simulink model "gm_UZ_EnDat"  (R2023b)
settings: Solver=FixedStepDiscrete  StartTime=0  StopTime=0.002  RelTol=1e-3
model workspace (MAT data in the model file):
  Select = 0
libraries: hdlsllib x314, hdlmdlgenlib x10, simulink x7, simulink_extras x3
(part 2 of 7)

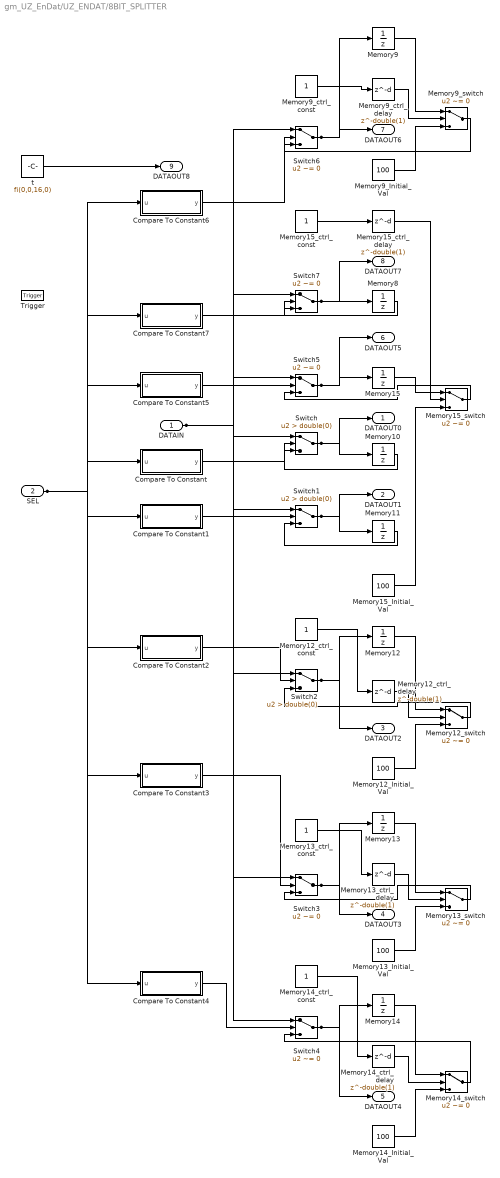
== system gm_UZ_EnDat/UZ_ENDAT/8BIT_SPLITTER ==
  DATAIN : Inport  OutDataTypeStr=uint16  PortDimensions=1
  SEL : Inport  Port=2  OutDataTypeStr=fixdt(0, 4, 0)  PortDimensions=1
  Trigger : TriggerPort  TriggerType=falling  VariantControl=(inherit)  OutputDataType=int8  InitialTriggerSignalState=positive  PortDimensions=1  OutDataTypeStr=boolean
  Compare To Constant : Subsystem  mask(Compare To Constant){relop===, const=double(0), OutDataTypeStr=boolean, ZeroCross=on}
      mask prompts: relop "Simulink:masks:Operator_MP"; const "Simulink:masks:ConstantValue_MP"; OutDataTypeStr "Simulink:masks:OutputDataType_MP"; ZeroCross "Simulink:masks:EnableZerocrossingDetection_MP"
      mask help: Simulink:masks:CompareToConstant_MD
      mask TypeOptions relop: == | ~= | < | <= | >= | >
      mask TypeOptions OutDataTypeStr: Simulink:masks:uint8 | Simulink:masks:boolean
      mask Callback ZeroCross: sl('zeroCrossEnable', gcbh);
      mask Display: disp(str)
  Compare To Constant1 : Subsystem  mask(Compare To Constant){relop===, const=double(1), OutDataTypeStr=boolean, ZeroCross=on}
      mask prompts: relop "Simulink:masks:Operator_MP"; const "Simulink:masks:ConstantValue_MP"; OutDataTypeStr "Simulink:masks:OutputDataType_MP"; ZeroCross "Simulink:masks:EnableZerocrossingDetection_MP"
      mask help: Simulink:masks:CompareToConstant_MD
      mask init:
      | OutDataTypeStr = 'boolean';
      | ZeroCross = 'on';
      | blkName = 'UZ_EnDat/UZ_ENDAT/8BIT_SPLITTER/Compare\nTo Constant1';
      | const = double(1);
      | const_str = '1';
      | const_val = double(1);
      | relop = '==';
      | setValue = 'boolean';
      | str = '== 1';
      mask TypeOptions relop: == | ~= | < | <= | >= | >
      mask TypeOptions OutDataTypeStr: Simulink:masks:uint8 | Simulink:masks:boolean
      mask Callback ZeroCross: sl('zeroCrossEnable', gcbh);
      mask Display: disp(str)
  Compare To Constant2 : Subsystem  mask(Compare To Constant){relop===, const=double(2), OutDataTypeStr=boolean, ZeroCross=on}
      mask prompts: relop "Simulink:masks:Operator_MP"; const "Simulink:masks:ConstantValue_MP"; OutDataTypeStr "Simulink:masks:OutputDataType_MP"; ZeroCross "Simulink:masks:EnableZerocrossingDetection_MP"
      mask help: Simulink:masks:CompareToConstant_MD
      mask init:
      | OutDataTypeStr = 'boolean';
      | ZeroCross = 'on';
      | blkName = 'UZ_EnDat/UZ_ENDAT/8BIT_SPLITTER/Compare\nTo Constant2';
      | const = double(2);
      | const_str = '2';
      | const_val = double(2);
      | relop = '==';
      | setValue = 'boolean';
      | str = '== 2';
      mask TypeOptions relop: == | ~= | < | <= | >= | >
      mask TypeOptions OutDataTypeStr: Simulink:masks:uint8 | Simulink:masks:boolean
      mask Callback ZeroCross: sl('zeroCrossEnable', gcbh);
      mask Display: disp(str)
  Compare To Constant3 : Subsystem  mask(Compare To Constant){relop===, const=double(3), OutDataTypeStr=boolean, ZeroCross=on}
      mask prompts: relop "Simulink:masks:Operator_MP"; const "Simulink:masks:ConstantValue_MP"; OutDataTypeStr "Simulink:masks:OutputDataType_MP"; ZeroCross "Simulink:masks:EnableZerocrossingDetection_MP"
      mask help: Simulink:masks:CompareToConstant_MD
      mask init:
      | OutDataTypeStr = 'boolean';
      | ZeroCross = 'on';
      | blkName = 'UZ_EnDat/UZ_ENDAT/8BIT_SPLITTER/Compare\nTo Constant3';
      | const = double(3);
      | const_str = '3';
      | const_val = double(3);
      | relop = '==';
      | setValue = 'boolean';
      | str = '== 3';
      mask TypeOptions relop: == | ~= | < | <= | >= | >
      mask TypeOptions OutDataTypeStr: Simulink:masks:uint8 | Simulink:masks:boolean
      mask Callback ZeroCross: sl('zeroCrossEnable', gcbh);
      mask Display: disp(str)
  Compare To Constant4 : Subsystem  mask(Compare To Constant){relop===, const=double(4), OutDataTypeStr=boolean, ZeroCross=on}
      mask prompts: relop "Simulink:masks:Operator_MP"; const "Simulink:masks:ConstantValue_MP"; OutDataTypeStr "Simulink:masks:OutputDataType_MP"; ZeroCross "Simulink:masks:EnableZerocrossingDetection_MP"
      mask help: Simulink:masks:CompareToConstant_MD
      mask init:
      | OutDataTypeStr = 'boolean';
      | ZeroCross = 'on';
      | blkName = 'UZ_EnDat/UZ_ENDAT/8BIT_SPLITTER/Compare\nTo Constant4';
      | const = double(4);
      | const_str = '4';
      | const_val = double(4);
      | relop = '==';
      | setValue = 'boolean';
      | str = '== 4';
      mask TypeOptions relop: == | ~= | < | <= | >= | >
      mask TypeOptions OutDataTypeStr: Simulink:masks:uint8 | Simulink:masks:boolean
      mask Callback ZeroCross: sl('zeroCrossEnable', gcbh);
      mask Display: disp(str)
  Compare To Constant5 : Subsystem  mask(Compare To Constant){relop===, const=double(5), OutDataTypeStr=boolean, ZeroCross=on}
      mask prompts: relop "Simulink:masks:Operator_MP"; const "Simulink:masks:ConstantValue_MP"; OutDataTypeStr "Simulink:masks:OutputDataType_MP"; ZeroCross "Simulink:masks:EnableZerocrossingDetection_MP"
      mask help: Simulink:masks:CompareToConstant_MD
      mask init:
      | OutDataTypeStr = 'boolean';
      | ZeroCross = 'on';
      | blkName = 'UZ_EnDat/UZ_ENDAT/8BIT_SPLITTER/Compare\nTo Constant5';
      | const = double(5);
      | const_str = '5';
      | const_val = double(5);
      | relop = '==';
      | setValue = 'boolean';
      | str = '== 5';
      mask TypeOptions relop: == | ~= | < | <= | >= | >
      mask TypeOptions OutDataTypeStr: Simulink:masks:uint8 | Simulink:masks:boolean
      mask Callback ZeroCross: sl('zeroCrossEnable', gcbh);
      mask Display: disp(str)
  Compare To Constant6 : Subsystem  mask(Compare To Constant){relop===, const=double(6), OutDataTypeStr=boolean, ZeroCross=on}
      mask prompts: relop "Simulink:masks:Operator_MP"; const "Simulink:masks:ConstantValue_MP"; OutDataTypeStr "Simulink:masks:OutputDataType_MP"; ZeroCross "Simulink:masks:EnableZerocrossingDetection_MP"
      mask help: Simulink:masks:CompareToConstant_MD
      mask init:
      | OutDataTypeStr = 'boolean';
      | ZeroCross = 'on';
      | blkName = 'UZ_EnDat/UZ_ENDAT/8BIT_SPLITTER/Compare\nTo Constant6';
      | const = double(6);
      | const_str = '6';
      | const_val = double(6);
      | relop = '==';
      | setValue = 'boolean';
      | str = '== 6';
      mask TypeOptions relop: == | ~= | < | <= | >= | >
      mask TypeOptions OutDataTypeStr: Simulink:masks:uint8 | Simulink:masks:boolean
      mask Callback ZeroCross: sl('zeroCrossEnable', gcbh);
      mask Display: disp(str)
  Compare To Constant7 : Subsystem  mask(Compare To Constant){relop===, const=double(7), OutDataTypeStr=boolean, ZeroCross=on}
      mask prompts: relop "Simulink:masks:Operator_MP"; const "Simulink:masks:ConstantValue_MP"; OutDataTypeStr "Simulink:masks:OutputDataType_MP"; ZeroCross "Simulink:masks:EnableZerocrossingDetection_MP"
      mask help: Simulink:masks:CompareToConstant_MD
      mask init:
      | OutDataTypeStr = 'boolean';
      | ZeroCross = 'on';
      | blkName = 'UZ_EnDat/UZ_ENDAT/8BIT_SPLITTER/Compare\nTo Constant7';
      | const = double(7);
      | const_str = '7';
      | const_val = double(7);
      | relop = '==';
      | setValue = 'boolean';
      | str = '== 7';
      mask TypeOptions relop: == | ~= | < | <= | >= | >
      mask TypeOptions OutDataTypeStr: Simulink:masks:uint8 | Simulink:masks:boolean
      mask Callback ZeroCross: sl('zeroCrossEnable', gcbh);
      mask Display: disp(str)
  Memory10 : UnitDelay  SampleTime=-1
  Memory11 : UnitDelay  SampleTime=-1
  Memory{9,12..15} (5 alike) : UnitDelay  InitialCondition=double(0)  SampleTime=-1
  Memory12_Initial_Val : Constant  Value=100  OutDataTypeStr=uint16  SampleTime=-1
  Memory12_ctrl_const : Constant  OutDataTypeStr=boolean  SampleTime=-1
  Memory12_ctrl_delay : Delay  DelayLength=double(1)  InitialCondition=0
  Memory12_switch : Switch  Criteria=u2 ~= 0  Threshold=double(0)  OutDataTypeStr=uint16  SaturateOnIntegerOverflow=off  InputSameDT=off
  Memory13_Initial_Val : Constant  Value=100  OutDataTypeStr=uint16  SampleTime=-1
  Memory13_ctrl_const : Constant  OutDataTypeStr=boolean  SampleTime=-1
  Memory13_ctrl_delay : Delay  DelayLength=double(1)  InitialCondition=0
  Memory13_switch : Switch  Criteria=u2 ~= 0  Threshold=double(0)  OutDataTypeStr=uint16  SaturateOnIntegerOverflow=off  InputSameDT=off
  Memory14_Initial_Val : Constant  Value=100  OutDataTypeStr=uint16  SampleTime=-1
  Memory14_ctrl_const : Constant  OutDataTypeStr=boolean  SampleTime=-1
  Memory14_ctrl_delay : Delay  DelayLength=double(1)  InitialCondition=0
  Memory14_switch : Switch  Criteria=u2 ~= 0  Threshold=double(0)  OutDataTypeStr=uint16  SaturateOnIntegerOverflow=off  InputSameDT=off
  Memory15_Initial_Val : Constant  Value=100  OutDataTypeStr=uint16  SampleTime=-1
  Memory15_ctrl_const : Constant  OutDataTypeStr=boolean  SampleTime=-1
  Memory15_ctrl_delay : Delay  DelayLength=double(1)  InitialCondition=0
  Memory15_switch : Switch  Criteria=u2 ~= 0  Threshold=double(0)  OutDataTypeStr=uint16  SaturateOnIntegerOverflow=off  InputSameDT=off
  Memory8 : UnitDelay  SampleTime=-1
  Memory9_Initial_Val : Constant  Value=100  OutDataTypeStr=uint16  SampleTime=-1
  Memory9_ctrl_const : Constant  OutDataTypeStr=boolean  SampleTime=-1
  Memory9_ctrl_delay : Delay  DelayLength=double(1)  InitialCondition=0
  Memory9_switch : Switch  Criteria=u2 ~= 0  Threshold=double(0)  OutDataTypeStr=uint16  SaturateOnIntegerOverflow=off  InputSameDT=off
  Switch : Switch  Criteria=u2 > Threshold  Threshold=double(0)  OutDataTypeStr=uint16  SaturateOnIntegerOverflow=off  InputSameDT=off
  Switch1 : Switch  Criteria=u2 > Threshold  Threshold=double(0)  OutDataTypeStr=uint16  SaturateOnIntegerOverflow=off  InputSameDT=off
  Switch2 : Switch  Criteria=u2 > Threshold  Threshold=double(0)  OutDataTypeStr=uint16  SaturateOnIntegerOverflow=off  InputSameDT=off
  Switch{3..6} (4 alike) : Switch  Criteria=u2 ~= 0  Threshold=double(0)  OutDataTypeStr=uint16  SaturateOnIntegerOverflow=off  InputSameDT=off
  Switch7 : Switch  Criteria=u2 ~= 0  Threshold=double(0)  OutDataTypeStr=int8  SaturateOnIntegerOverflow=off  InputSameDT=off
  t : Constant  Value=fi(0,0,16,0)  OutDataTypeStr=uint16  SampleTime=-1
  DATAOUT0 : Outport  InitialOutput=0
  DATAOUT1 : Outport  Port=2  InitialOutput=0
  DATAOUT2 : Outport  Port=3  InitialOutput=0
  DATAOUT3 : Outport  Port=4  InitialOutput=0
  DATAOUT4 : Outport  Port=5  InitialOutput=0
  DATAOUT5 : Outport  Port=6  InitialOutput=0
  DATAOUT6 : Outport  Port=7  InitialOutput=0
  DATAOUT7 : Outport  Port=8  InitialOutput=0
  DATAOUT8 : Outport  Port=9  InitialOutput=0
  wires:
  DATAIN/1 -> Switch/1, Switch1/1, Switch2/1, Switch3/1, Switch4/1, Switch5/1, Switch6/1, Switch7/1
  SEL/1 -> Compare To Constant6/1(u), Compare To Constant7/1(u), Compare To Constant5/1(u), Compare To Constant4/1(u), Compare To Constant2/1(u), Compare To Constant1/1(u), Compare To Constant/1(u), Compare To Constant3/1(u)
  Switch/1 -> DATAOUT0/1, Memory10/1
  Switch1/1 -> DATAOUT1/1, Memory11/1
  Switch2/1 -> DATAOUT2/1, Memory12/1
  Switch3/1 -> DATAOUT3/1, Memory13/1
  Switch4/1 -> DATAOUT4/1, Memory14/1
  Switch5/1 -> DATAOUT5/1, Memory15/1
  Switch6/1 -> DATAOUT6/1, Memory9/1
  Switch7/1 -> DATAOUT7/1, Memory8/1
  t/1 -> DATAOUT8/1
  Compare To Constant7/1(y) -> Switch7/2
  Memory8/1 -> Switch7/3
  Compare To Constant/1(y) -> Switch/2
  Memory10/1 -> Switch/3
  Compare To Constant1/1(y) -> Switch1/2
  Memory11/1 -> Switch1/3
  Memory12/1 -> Memory12_switch/1
  Memory12_ctrl_delay/1 -> Memory12_switch/2
  Memory12_Initial_Val/1 -> Memory12_switch/3
  Compare To Constant2/1(y) -> Switch2/2
  Memory12_switch/1 -> Switch2/3
  Memory13/1 -> Memory13_switch/1
  Memory13_ctrl_delay/1 -> Memory13_switch/2
  Memory13_Initial_Val/1 -> Memory13_switch/3
  Compare To Constant3/1(y) -> Switch3/2
  Memory13_switch/1 -> Switch3/3
  Memory14/1 -> Memory14_switch/1
  Memory14_ctrl_delay/1 -> Memory14_switch/2
  Memory14_Initial_Val/1 -> Memory14_switch/3
  Compare To Constant4/1(y) -> Switch4/2
  Memory14_switch/1 -> Switch4/3
  Memory15/1 -> Memory15_switch/1
  Memory15_ctrl_delay/1 -> Memory15_switch/2
  Memory15_Initial_Val/1 -> Memory15_switch/3
  Compare To Constant5/1(y) -> Switch5/2
  Memory15_switch/1 -> Switch5/3
  Memory9/1 -> Memory9_switch/1
  Memory9_ctrl_delay/1 -> Memory9_switch/2
  Memory9_Initial_Val/1 -> Memory9_switch/3
  Compare To Constant6/1(y) -> Switch6/2
  Memory9_switch/1 -> Switch6/3
  Memory12_ctrl_const/1 -> Memory12_ctrl_delay/1
  Memory13_ctrl_const/1 -> Memory13_ctrl_delay/1
  Memory14_ctrl_const/1 -> Memory14_ctrl_delay/1
  Memory15_ctrl_const/1 -> Memory15_ctrl_delay/1
  Memory9_ctrl_const/1 -> Memory9_ctrl_delay/1

== system gm_UZ_EnDat/UZ_ENDAT/CLKCNTER_ACT ==
  CLK : Inport  OutDataTypeStr=boolean  PortDimensions=1  SampleTime=1e-08
  CLK2CNT : Inport  Port=2  OutDataTypeStr=boolean  PortDimensions=1  SampleTime=1e-08
  ResetCNT : Inport  Port=3  OutDataTypeStr=boolean  PortDimensions=1  SampleTime=1e-08
  Delay1 : Delay  DelayLength=double(1)  InitialCondition=0  SampleTime=1e-08
  Positional_Counter : Subsystem
  SetZero32modified : Subsystem
  CNT : Outport  SampleTime=1e-08
  wires:
  Positional_Counter/1(divider) -> SetZero32modified/1(valin)
  CLK/1 -> SetZero32modified/Trigger
  ResetCNT/1 -> SetZero32modified/2(setzero)
  CLK2CNT/1 -> Positional_Counter/Trigger
  SetZero32modified/1(valueout) -> Delay1/1
  Delay1/1 -> Positional_Counter/1(valueout), CNT/1

== system gm_UZ_EnDat/UZ_ENDAT/CLKCNTER_NOSTOP ==
  CLK : Inport  OutDataTypeStr=boolean  PortDimensions=1  SampleTime=1e-08
  CLK2CNT : Inport  Port=2  OutDataTypeStr=boolean  PortDimensions=1  SampleTime=1e-08
  ResetCNT : Inport  Port=3  OutDataTypeStr=boolean  PortDimensions=1  SampleTime=1e-08
  Delay1 : Delay  DelayLength=double(1)  InitialCondition=0  SampleTime=1e-08
  Positional_Counter : Subsystem
  SetZero32modified : Subsystem
  CNT : Outport  SampleTime=1e-08
  wires:
  Delay1/1 -> CNT/1, Positional_Counter/1(valueout)
  SetZero32modified/1(valueout) -> Delay1/1
  CLK2CNT/1 -> Positional_Counter/Trigger
  ResetCNT/1 -> SetZero32modified/2(setzero)
  CLK/1 -> SetZero32modified/Trigger
  Positional_Counter/1(divider) -> SetZero32modified/1(valin)

== system gm_UZ_EnDat/UZ_ENDAT/CLKDIV1 ==
  CLK1 : Inport  OutDataTypeStr=boolean  PortDimensions=1  SampleTime=1e-08
  Delay : Delay  DelayLength=double(1)  InitialCondition=0  SampleTime=1e-08
  Logical Operator1 : Logic  Operator=NOT  Inputs=1  AllPortsSameDT=off  OutDataTypeStr=boolean  SampleTime=1e-08
  Triggered Subsystem : Subsystem
  CLK/2 : Outport  OutDataTypeStr=boolean  SampleTime=1e-08  VectorParamsAs1DForOutWhenUnconnected=off
  wires:
  Logical Operator1/1 -> CLK/2/1, Delay/1
  Delay/1 -> Triggered Subsystem/1(IN)
  CLK1/1 -> Triggered Subsystem/Trigger
  Triggered Subsystem/1(OUT) -> Logical Operator1/1

== system gm_UZ_EnDat/UZ_ENDAT/CLKDIV3 ==
  CLK1 : Inport  OutDataTypeStr=boolean  PortDimensions=1  SampleTime=1e-08
  Delay : Delay  DelayLength=double(1)  InitialCondition=0  SampleTime=1e-08
  Logical Operator1 : Logic  Operator=NOT  Inputs=1  AllPortsSameDT=off  OutDataTypeStr=boolean  SampleTime=1e-08
  Triggered Subsystem : Subsystem
  CLK/2 : Outport  OutDataTypeStr=boolean  SampleTime=1e-08  VectorParamsAs1DForOutWhenUnconnected=off
  wires:
  Triggered Subsystem/1(OUT) -> Logical Operator1/1
  CLK1/1 -> Triggered Subsystem/Trigger
  Delay/1 -> Triggered Subsystem/1(IN)
  Logical Operator1/1 -> Delay/1, CLK/2/1

== system gm_UZ_EnDat/UZ_ENDAT/CLKDIV4 ==
  CLK1 : Inport  OutDataTypeStr=boolean  PortDimensions=1  SampleTime=1e-08
  Delay : Delay  DelayLength=double(1)  InitialCondition=0  SampleTime=1e-08
  Logical Operator1 : Logic  Operator=NOT  Inputs=1  AllPortsSameDT=off  OutDataTypeStr=boolean  SampleTime=1e-08
  Triggered Subsystem : Subsystem
  CLK/2 : Outport  OutDataTypeStr=boolean  SampleTime=1e-08  VectorParamsAs1DForOutWhenUnconnected=off
  wires:
  Triggered Subsystem/1(OUT) -> Logical Operator1/1
  CLK1/1 -> Triggered Subsystem/Trigger
  Delay/1 -> Triggered Subsystem/1(IN)
  Logical Operator1/1 -> Delay/1, CLK/2/1

== system gm_UZ_EnDat/UZ_ENDAT/CLKDIV5 ==
  CLK1 : Inport  OutDataTypeStr=boolean  PortDimensions=1  SampleTime=1e-08
  Delay : Delay  DelayLength=double(1)  InitialCondition=0  SampleTime=1e-08
  Logical Operator1 : Logic  Operator=NOT  Inputs=1  AllPortsSameDT=off  OutDataTypeStr=boolean  SampleTime=1e-08
  Triggered Subsystem : Subsystem
  CLK/2 : Outport  OutDataTypeStr=boolean  SampleTime=1e-08  VectorParamsAs1DForOutWhenUnconnected=off
  wires:
  Triggered Subsystem/1(OUT) -> Logical Operator1/1
  CLK1/1 -> Triggered Subsystem/Trigger
  Delay/1 -> Triggered Subsystem/1(IN)
  Logical Operator1/1 -> Delay/1, CLK/2/1

== system gm_UZ_EnDat/UZ_ENDAT/CLKDIV6 ==
  CLK1 : Inport  OutDataTypeStr=boolean  PortDimensions=1  SampleTime=1e-08
  Delay : Delay  DelayLength=double(1)  InitialCondition=0  SampleTime=1e-08
  Logical Operator1 : Logic  Operator=NOT  Inputs=1  AllPortsSameDT=off  OutDataTypeStr=boolean  SampleTime=1e-08
  Triggered Subsystem : Subsystem
  CLK/2 : Outport  OutDataTypeStr=boolean  SampleTime=1e-08  VectorParamsAs1DForOutWhenUnconnected=off
  wires:
  Triggered Subsystem/1(OUT) -> Logical Operator1/1
  CLK1/1 -> Triggered Subsystem/Trigger
  Delay/1 -> Triggered Subsystem/1(IN)
  Logical Operator1/1 -> Delay/1, CLK/2/1

== system gm_UZ_EnDat/UZ_ENDAT/CLKDIV7 ==
  CLK1 : Inport  OutDataTypeStr=boolean  PortDimensions=1  SampleTime=1e-08
  Delay : Delay  DelayLength=double(1)  InitialCondition=0  SampleTime=1e-08
  Logical Operator1 : Logic  Operator=NOT  Inputs=1  AllPortsSameDT=off  OutDataTypeStr=boolean  SampleTime=1e-08
  Triggered Subsystem : Subsystem
  CLK/2 : Outport  OutDataTypeStr=boolean  SampleTime=1e-08  VectorParamsAs1DForOutWhenUnconnected=off
  wires:
  Triggered Subsystem/1(OUT) -> Logical Operator1/1
  CLK1/1 -> Triggered Subsystem/Trigger
  Delay/1 -> Triggered Subsystem/1(IN)
  Logical Operator1/1 -> Delay/1, CLK/2/1

== system gm_UZ_EnDat/UZ_ENDAT/CLKDIV8 ==
  CLK1 : Inport  OutDataTypeStr=boolean  PortDimensions=1  SampleTime=1e-08
  Delay : Delay  DelayLength=double(1)  InitialCondition=0  SampleTime=1e-08
  Logical Operator1 : Logic  Operator=NOT  Inputs=1  AllPortsSameDT=off  OutDataTypeStr=boolean  SampleTime=1e-08
  Triggered Subsystem : Subsystem
  CLK/2 : Outport  OutDataTypeStr=boolean  SampleTime=1e-08  VectorParamsAs1DForOutWhenUnconnected=off
  wires:
  Triggered Subsystem/1(OUT) -> Logical Operator1/1
  CLK1/1 -> Triggered Subsystem/Trigger
  Delay/1 -> Triggered Subsystem/1(IN)
  Logical Operator1/1 -> Delay/1, CLK/2/1

== system gm_UZ_EnDat/UZ_ENDAT/CLKDIV9 ==
  CLK1 : Inport  OutDataTypeStr=boolean  PortDimensions=1  SampleTime=1e-08
  Delay : Delay  DelayLength=double(1)  InitialCondition=0  SampleTime=1e-08
  Logical Operator1 : Logic  Operator=NOT  Inputs=1  AllPortsSameDT=off  OutDataTypeStr=boolean  SampleTime=1e-08
  Triggered Subsystem : Subsystem
  CLK/2 : Outport  OutDataTypeStr=boolean  SampleTime=1e-08  VectorParamsAs1DForOutWhenUnconnected=off
  wires:
  Triggered Subsystem/1(OUT) -> Logical Operator1/1
  CLK1/1 -> Triggered Subsystem/Trigger
  Delay/1 -> Triggered Subsystem/1(IN)
  Logical Operator1/1 -> Delay/1, CLK/2/1

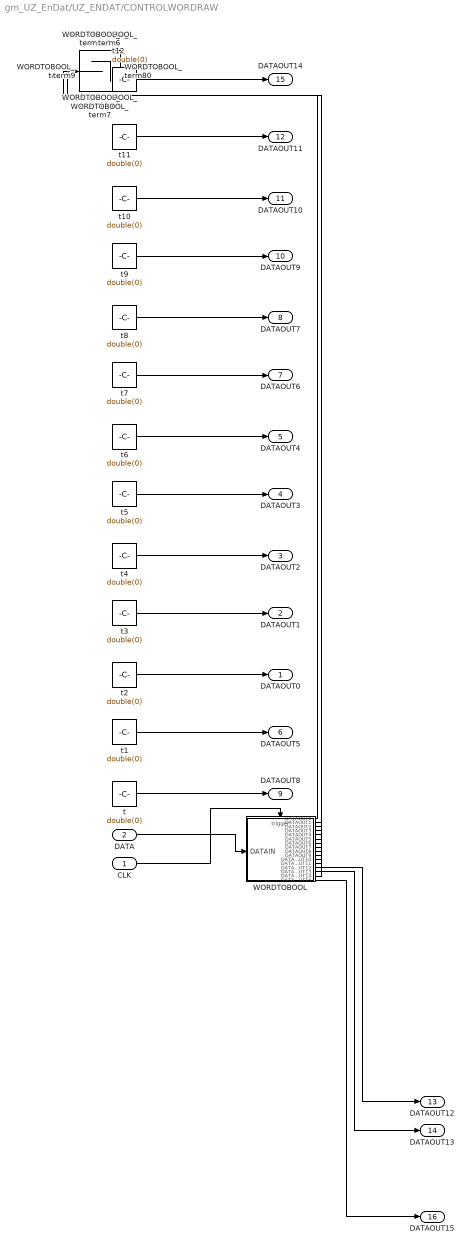
== system gm_UZ_EnDat/UZ_ENDAT/CONTROLWORDRAW ==
  CLK : Inport  OutDataTypeStr=boolean  PortDimensions=1  SampleTime=1e-08
  DATA : Inport  Port=2  OutDataTypeStr=uint16  PortDimensions=1  SampleTime=1e-08
  WORDTOBOOL : Subsystem
  WORDTOBOOL_term{0..11,14} (13 alike) : Terminator
  t{,1..12} (13 alike) : Constant  Value=double(0)  OutDataTypeStr=boolean  SampleTime=1e-08
  DATAOUT0 : Outport  SampleTime=1e-08  VectorParamsAs1DForOutWhenUnconnected=off
  DATAOUT1 : Outport  Port=2  SampleTime=1e-08  VectorParamsAs1DForOutWhenUnconnected=off
  DATAOUT2 : Outport  Port=3  SampleTime=1e-08  VectorParamsAs1DForOutWhenUnconnected=off
  DATAOUT3 : Outport  Port=4  SampleTime=1e-08  VectorParamsAs1DForOutWhenUnconnected=off
  DATAOUT4 : Outport  Port=5  SampleTime=1e-08  VectorParamsAs1DForOutWhenUnconnected=off
  DATAOUT5 : Outport  Port=6  SampleTime=1e-08  VectorParamsAs1DForOutWhenUnconnected=off
  DATAOUT6 : Outport  Port=7  SampleTime=1e-08  VectorParamsAs1DForOutWhenUnconnected=off
  DATAOUT7 : Outport  Port=8  SampleTime=1e-08  VectorParamsAs1DForOutWhenUnconnected=off
  DATAOUT8 : Outport  Port=9  SampleTime=1e-08  VectorParamsAs1DForOutWhenUnconnected=off
  DATAOUT9 : Outport  Port=10  SampleTime=1e-08  VectorParamsAs1DForOutWhenUnconnected=off
  DATAOUT10 : Outport  Port=11  SampleTime=1e-08  VectorParamsAs1DForOutWhenUnconnected=off
  DATAOUT11 : Outport  Port=12  SampleTime=1e-08  VectorParamsAs1DForOutWhenUnconnected=off
  DATAOUT12 : Outport  Port=13  SampleTime=1e-08  VectorParamsAs1DForOutWhenUnconnected=off
  DATAOUT13 : Outport  Port=14  SampleTime=1e-08  VectorParamsAs1DForOutWhenUnconnected=off
  DATAOUT14 : Outport  Port=15  SampleTime=1e-08  VectorParamsAs1DForOutWhenUnconnected=off
  DATAOUT15 : Outport  Port=16  SampleTime=1e-08  VectorParamsAs1DForOutWhenUnconnected=off
  wires:
  CLK/1 -> WORDTOBOOL/Trigger
  DATA/1 -> WORDTOBOOL/1(DATAIN)
  t2/1 -> DATAOUT0/1
  t3/1 -> DATAOUT1/1
  t4/1 -> DATAOUT2/1
  t5/1 -> DATAOUT3/1
  t6/1 -> DATAOUT4/1
  t1/1 -> DATAOUT5/1
  t7/1 -> DATAOUT6/1
  t8/1 -> DATAOUT7/1
  t/1 -> DATAOUT8/1
  t9/1 -> DATAOUT9/1
  t10/1 -> DATAOUT10/1
  t11/1 -> DATAOUT11/1
  WORDTOBOOL/13(DATAOUT12) -> DATAOUT12/1
  WORDTOBOOL/14(DATAOUT13) -> DATAOUT13/1
  t12/1 -> DATAOUT14/1
  WORDTOBOOL/16(DATAOUT15) -> DATAOUT15/1
  WORDTOBOOL/1(DATAOUT0) -> WORDTOBOOL_term0/1
  WORDTOBOOL/2(DATAOUT1) -> WORDTOBOOL_term1/1
  WORDTOBOOL/3(DATAOUT2) -> WORDTOBOOL_term2/1
  WORDTOBOOL/4(DATAOUT3) -> WORDTOBOOL_term3/1
  WORDTOBOOL/5(DATAOUT4) -> WORDTOBOOL_term4/1
  WORDTOBOOL/6(DATAOUT5) -> WORDTOBOOL_term5/1
  WORDTOBOOL/7(DATAOUT6) -> WORDTOBOOL_term6/1
  WORDTOBOOL/8(DATAOUT7) -> WORDTOBOOL_term7/1
  WORDTOBOOL/9(DATAOUT8) -> WORDTOBOOL_term8/1
  WORDTOBOOL/10(DATAOUT9) -> WORDTOBOOL_term9/1
  WORDTOBOOL/11(DATAOUT10) -> WORDTOBOOL_term10/1
  WORDTOBOOL/12(DATAOUT11) -> WORDTOBOOL_term11/1
  WORDTOBOOL/15(DATAOUT14) -> WORDTOBOOL_term14/1

== system gm_UZ_EnDat/UZ_ENDAT/CONTROLWORDSTORED ==
  CLK : Inport  OutDataTypeStr=boolean  PortDimensions=1  SampleTime=1e-08
  DATA : Inport  Port=2  OutDataTypeStr=uint16  PortDimensions=1  SampleTime=1e-08
  WORDTOBOOL : Subsystem
  WORDTOBOOL_term13 : Terminator
  t : Constant  Value=double(0)  OutDataTypeStr=boolean  SampleTime=1e-08
  DATAOUT0 : Outport  SampleTime=1e-08  VectorParamsAs1DForOutWhenUnconnected=off
  DATAOUT1 : Outport  Port=2  SampleTime=1e-08  VectorParamsAs1DForOutWhenUnconnected=off
  DATAOUT2 : Outport  Port=3  SampleTime=1e-08  VectorParamsAs1DForOutWhenUnconnected=off
  DATAOUT3 : Outport  Port=4  SampleTime=1e-08  VectorParamsAs1DForOutWhenUnconnected=off
  DATAOUT4 : Outport  Port=5  SampleTime=1e-08  VectorParamsAs1DForOutWhenUnconnected=off
  DATAOUT5 : Outport  Port=6  SampleTime=1e-08  VectorParamsAs1DForOutWhenUnconnected=off
  DATAOUT6 : Outport  Port=7  SampleTime=1e-08  VectorParamsAs1DForOutWhenUnconnected=off
  DATAOUT7 : Outport  Port=8  SampleTime=1e-08  VectorParamsAs1DForOutWhenUnconnected=off
  DATAOUT8 : Outport  Port=9  SampleTime=1e-08  VectorParamsAs1DForOutWhenUnconnected=off
  DATAOUT9 : Outport  Port=10  SampleTime=1e-08  VectorParamsAs1DForOutWhenUnconnected=off
  DATAOUT10 : Outport  Port=11  SampleTime=1e-08  VectorParamsAs1DForOutWhenUnconnected=off
  DATAOUT11 : Outport  Port=12  SampleTime=1e-08  VectorParamsAs1DForOutWhenUnconnected=off
  DATAOUT12 : Outport  Port=13  SampleTime=1e-08  VectorParamsAs1DForOutWhenUnconnected=off
  DATAOUT13 : Outport  Port=14  SampleTime=1e-08  VectorParamsAs1DForOutWhenUnconnected=off
  DATAOUT14 : Outport  Port=15  SampleTime=1e-08  VectorParamsAs1DForOutWhenUnconnected=off
  DATAOUT15 : Outport  Port=16  SampleTime=1e-08  VectorParamsAs1DForOutWhenUnconnected=off
  wires:
  CLK/1 -> WORDTOBOOL/Trigger
  DATA/1 -> WORDTOBOOL/1(DATAIN)
  WORDTOBOOL/1(DATAOUT0) -> DATAOUT0/1
  WORDTOBOOL/2(DATAOUT1) -> DATAOUT1/1
  WORDTOBOOL/3(DATAOUT2) -> DATAOUT2/1
  WORDTOBOOL/4(DATAOUT3) -> DATAOUT3/1
  WORDTOBOOL/5(DATAOUT4) -> DATAOUT4/1
  WORDTOBOOL/6(DATAOUT5) -> DATAOUT5/1
  WORDTOBOOL/7(DATAOUT6) -> DATAOUT6/1
  WORDTOBOOL/8(DATAOUT7) -> DATAOUT7/1
  WORDTOBOOL/9(DATAOUT8) -> DATAOUT8/1
  WORDTOBOOL/10(DATAOUT9) -> DATAOUT9/1
  WORDTOBOOL/11(DATAOUT10) -> DATAOUT10/1
  WORDTOBOOL/12(DATAOUT11) -> DATAOUT11/1
  WORDTOBOOL/13(DATAOUT12) -> DATAOUT12/1
  t/1 -> DATAOUT13/1
  WORDTOBOOL/15(DATAOUT14) -> DATAOUT14/1
  WORDTOBOOL/16(DATAOUT15) -> DATAOUT15/1
  WORDTOBOOL/14(DATAOUT13) -> WORDTOBOOL_term13/1

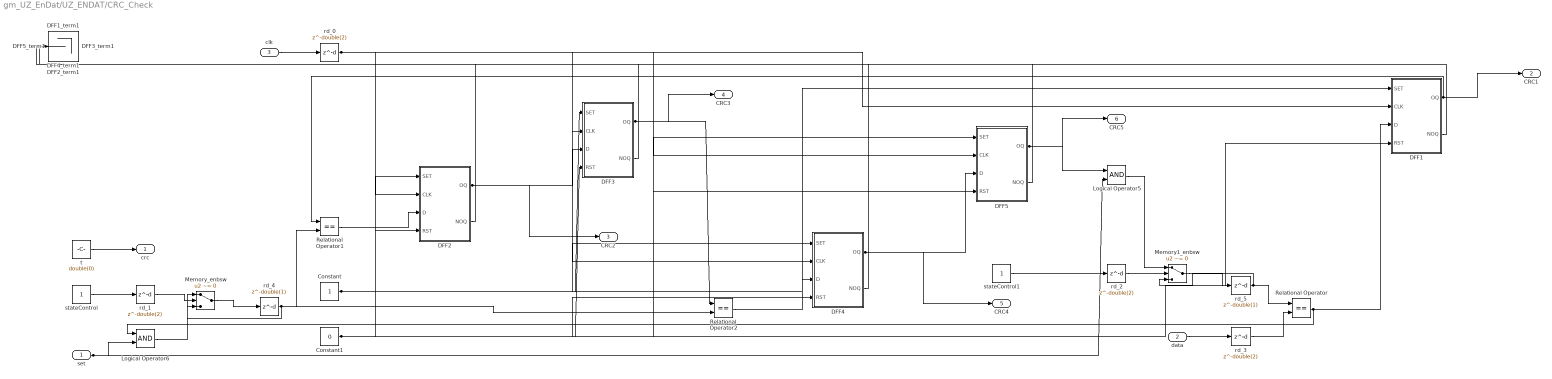
== system gm_UZ_EnDat/UZ_ENDAT/CRC_Check ==
  set : Inport  OutDataTypeStr=boolean  PortDimensions=1  SampleTime=1e-08
  data : Inport  Port=2  OutDataTypeStr=boolean  PortDimensions=1  SampleTime=1e-08
  clk : Inport  Port=3  OutDataTypeStr=boolean  PortDimensions=1  SampleTime=1e-08
  Constant : Constant  OutDataTypeStr=boolean  SampleTime=1e-08
  Constant1 : Constant  Value=0  OutDataTypeStr=boolean  SampleTime=1e-08
  DFF1 : Subsystem
  DFF1_term1 : Terminator
  DFF2 : Subsystem
  DFF2_term1 : Terminator
  DFF3 : Subsystem
  DFF3_term1 : Terminator
  DFF4 : Subsystem
  DFF4_term1 : Terminator
  DFF5 : Subsystem
  DFF5_term1 : Terminator
  Logical Operator5 : Logic  AllPortsSameDT=off  OutDataTypeStr=boolean  SampleTime=1e-08
  Logical Operator6 : Logic  AllPortsSameDT=off  OutDataTypeStr=boolean  SampleTime=1e-08
  Memory1_enbsw : Switch  Criteria=u2 ~= 0  Threshold=double(0)  OutDataTypeStr=boolean  SampleTime=1e-08  SaturateOnIntegerOverflow=off  InputSameDT=off
  Memory_enbsw : Switch  Criteria=u2 ~= 0  Threshold=double(0)  OutDataTypeStr=boolean  SampleTime=1e-08  SaturateOnIntegerOverflow=off  InputSameDT=off
  Relational Operator : RelationalOperator  Operator===  OutDataTypeStr=boolean  SampleTime=1e-08  InputSameDT=off
  Relational Operator1 : RelationalOperator  Operator===  OutDataTypeStr=boolean  SampleTime=1e-08  InputSameDT=off
  Relational Operator2 : RelationalOperator  Operator===  OutDataTypeStr=boolean  SampleTime=1e-08  InputSameDT=off
  rd_{0..3} (4 alike) : Delay  DelayLength=double(2)  InitialCondition=0  SampleTime=1e-08
  rd_4 : Delay  DelayLength=double(1)  InitialCondition=0  SampleTime=1e-08
  rd_5 : Delay  DelayLength=double(1)  InitialCondition=0  SampleTime=1e-08
  stateControl : Constant  OutDataTypeStr=boolean  SampleTime=1e-08
  stateControl1 : Constant  OutDataTypeStr=boolean  SampleTime=1e-08
  t : Constant  Value=double(0)  OutDataTypeStr=boolean  SampleTime=1e-08
  crc : Outport  SampleTime=1e-08
  CRC1 : Outport  Port=2  SampleTime=1e-08
  CRC2 : Outport  Port=3  SampleTime=1e-08
  CRC3 : Outport  Port=4  SampleTime=1e-08
  CRC4 : Outport  Port=5  SampleTime=1e-08
  CRC5 : Outport  Port=6  SampleTime=1e-08
  wires:
  set/1 -> Logical Operator5/2, Logical Operator6/2
  Constant/1 -> DFF4/1(SET), DFF5/1(SET), DFF1/1(SET), DFF2/1(SET), DFF3/1(SET)
  Constant1/1 -> DFF4/4(RST), DFF5/4(RST), DFF1/4(RST), DFF2/4(RST), DFF3/4(RST)
  t/1 -> crc/1
  data/1 -> rd_3/1
  stateControl/1 -> rd_1/1
  stateControl1/1 -> rd_2/1
  DFF2/1(OQ) -> DFF3/3(D), CRC2/1
  DFF2/2(NOQ) -> DFF2_term1/1
  DFF3/1(OQ) -> Relational Operator2/1, CRC3/1
  DFF3/2(NOQ) -> DFF3_term1/1
  DFF4/1(OQ) -> DFF5/3(D), CRC4/1
  DFF4/2(NOQ) -> DFF4_term1/1
  DFF5/1(OQ) -> Logical Operator5/1, CRC5/1
  DFF5/2(NOQ) -> DFF5_term1/1
  DFF1/1(OQ) -> Relational Operator1/1, CRC1/1
  DFF1/2(NOQ) -> DFF1_term1/1
  Relational Operator/1 -> DFF1/3(D), Logical Operator6/1
  Relational Operator2/1 -> DFF4/3(D)
  Relational Operator1/1 -> DFF2/3(D)
  Logical Operator6/1 -> Memory_enbsw/1
  Logical Operator5/1 -> Memory1_enbsw/1
  rd_1/1 -> Memory_enbsw/2
  rd_2/1 -> Memory1_enbsw/2
  rd_3/1 -> Relational Operator/2
  clk/1 -> rd_0/1
  rd_0/1 -> DFF3/2(CLK), DFF2/2(CLK), DFF1/2(CLK), DFF5/2(CLK), DFF4/2(CLK)
  Memory_enbsw/1 -> rd_4/1
  rd_4/1 -> Memory_enbsw/3, Relational Operator2/2, Relational Operator1/2
  Memory1_enbsw/1 -> rd_5/1
  rd_5/1 -> Memory1_enbsw/3, Relational Operator/1

== system gm_UZ_EnDat/UZ_ENDAT/Compare To Constant ==
  u : Inport  OutDataTypeStr=fixdt(0, 4, 0)  SampleTime=1e-08
  Compare : RelationalOperator  Operator===  OutDataTypeStr=boolean
  Constant : Constant  DisableCoverage=on  Value=const  OutDataTypeStr=Inherit: Inherit via back propagation  SampleTime=-1
  y : Outport  SampleTime=1e-08
  wires:
  u/1 -> Compare/1
  Compare/1 -> y/1
  Constant/1 -> Compare/2

== system gm_UZ_EnDat/UZ_ENDAT/Compare To Constant1 ==
  u : Inport  OutDataTypeStr=fixdt(0, 4, 0)  SampleTime=1e-08
  Compare : RelationalOperator  Operator===  OutDataTypeStr=boolean
  Constant : Constant  DisableCoverage=on  Value=const  OutDataTypeStr=Inherit: Inherit via back propagation  SampleTime=-1
  y : Outport  SampleTime=1e-08
  wires:
  u/1 -> Compare/1
  Compare/1 -> y/1
  Constant/1 -> Compare/2

== system gm_UZ_EnDat/UZ_ENDAT/Compare To Constant2 ==
  u : Inport  OutDataTypeStr=fixdt(0, 4, 0)  SampleTime=1e-08
  Compare : RelationalOperator  Operator===  OutDataTypeStr=boolean  SampleTime=1e-08
  Constant : Constant  Value=0  OutDataTypeStr=fixdt(0, 4, 0)  SampleTime=1e-08
  y : Outport  SampleTime=1e-08
  wires:
  u/1 -> Compare/1
  Compare/1 -> y/1
  Constant/1 -> Compare/2

== system gm_UZ_EnDat/UZ_ENDAT/Compare To Constant3 ==
  u : Inport  OutDataTypeStr=uint32  SampleTime=1e-08
  Compare : RelationalOperator  OutDataTypeStr=boolean
  Constant : Constant  DisableCoverage=on  Value=const  OutDataTypeStr=Inherit: Inherit via back propagation  SampleTime=-1
  y : Outport  SampleTime=1e-08
  wires:
  u/1 -> Compare/1
  Compare/1 -> y/1
  Constant/1 -> Compare/2

== system gm_UZ_EnDat/UZ_ENDAT/DATA2CLOCKSYNCER ==
  In1 : Inport  OutDataTypeStr=fixdt(0, 4, 0)  PortDimensions=1  SampleTime=1e-08
  FAKTOR : Inport  Port=2  OutDataTypeStr=uint16  PortDimensions=1  SampleTime=1e-08
  Constant : Constant  Value=100  OutDataTypeStr=uint16  SampleTime=1e-08
  Constant1 : Constant  Value=45  OutDataTypeStr=uint16  SampleTime=1e-08
  Constant2 : Constant  Value=2  OutDataTypeStr=uint16  SampleTime=1e-08
  Constant23 : Constant  Value=20  OutDataTypeStr=uint16  SampleTime=1e-08
  Constant24 : Constant  Value=29  OutDataTypeStr=uint16  SampleTime=1e-08
  Constant3 : Constant  Value=12  OutDataTypeStr=uint16  SampleTime=1e-08
  Constant4 : Constant  Value=4  OutDataTypeStr=uint16  SampleTime=1e-08
  Constant7 : Constant  Value=8  OutDataTypeStr=uint16  SampleTime=1e-08
  Divide : Product  Inputs=*/  OutDataTypeStr=uint16  RndMeth=Simplest  SaturateOnIntegerOverflow=on  SampleTime=1e-08
  HwModeRegister : Delay  DelayLength=double(1)  InitialCondition=0  SampleTime=1e-08
  HwModeRegister1 : Delay  DelayLength=double(1)  InitialCondition=0  SampleTime=1e-08
  Multiport Switch1 : MultiPortSwitch  DataPortOrder=Zero-based contiguous  Inputs=7  DiagnosticForDefault=None  zeroidx=on  OutDataTypeStr=uint16  SampleTime=1e-08  SaturateOnIntegerOverflow=off  InputSameDT=off
  PipelineRegister : Delay  DelayLength=double(1)  InitialCondition=0  SampleTime=1e-08
  Product : Product  Inputs=**  OutDataTypeStr=uint32  SampleTime=1e-08
  Product_out_dtc : DataTypeConversion  OutDataTypeStr=uint16  RndMeth=Simplest  SampleTime=1e-08
  Out1 : Outport  SampleTime=1e-08
  wires:
  In1/1 -> Multiport Switch1/1
  FAKTOR/1 -> HwModeRegister1/1
  Constant/1 -> Divide/2
  Constant1/1 -> Multiport Switch1/8
  Constant2/1 -> Multiport Switch1/2
  Constant23/1 -> Multiport Switch1/6
  Constant24/1 -> Multiport Switch1/7
  Constant3/1 -> Multiport Switch1/5
  Constant4/1 -> Multiport Switch1/3
  Constant7/1 -> Multiport Switch1/4
  Divide/1 -> Out1/1
  Multiport Switch1/1 -> HwModeRegister/1
  Product_out_dtc/1 -> Divide/1
  PipelineRegister/1 -> Product_out_dtc/1
  Product/1 -> PipelineRegister/1
  HwModeRegister/1 -> Product/1
  HwModeRegister1/1 -> Product/2

== system gm_UZ_EnDat/UZ_ENDAT/DATAFLOWCHGER ==
  CLKSEL : Inport  OutDataTypeStr=fixdt(0, 4, 0)  PortDimensions=1  SampleTime=1e-08
  FACTOR : Inport  Port=2  OutDataTypeStr=uint16  PortDimensions=1  SampleTime=1e-08
  Constant : Constant  Value=100  OutDataTypeStr=uint16  SampleTime=1e-08
  Constant{14..18,27..28} (7 alike) : Constant  Value=10  OutDataTypeStr=uint16  SampleTime=1e-08
  Divide : Product  Inputs=*/  OutDataTypeStr=uint16  RndMeth=Simplest  SaturateOnIntegerOverflow=on  SampleTime=1e-08
  HwModeRegister : Delay  DelayLength=double(1)  InitialCondition=0  SampleTime=1e-08
  HwModeRegister1 : Delay  DelayLength=double(1)  InitialCondition=0  SampleTime=1e-08
  Multiport Switch2 : MultiPortSwitch  DataPortOrder=Zero-based contiguous  Inputs=7  DiagnosticForDefault=None  zeroidx=on  OutDataTypeStr=uint16  SampleTime=1e-08  SaturateOnIntegerOverflow=off  InputSameDT=off
  PipelineRegister : Delay  DelayLength=double(1)  InitialCondition=0  SampleTime=1e-08
  Product : Product  Inputs=**  OutDataTypeStr=uint32  SampleTime=1e-08
  Product_out_dtc : DataTypeConversion  OutDataTypeStr=uint16  RndMeth=Simplest  SampleTime=1e-08
  Output : Outport  SampleTime=1e-08
  wires:
  CLKSEL/1 -> Multiport Switch2/1
  FACTOR/1 -> HwModeRegister1/1
  Constant/1 -> Divide/2
  Constant14/1 -> Multiport Switch2/8
  Constant15/1 -> Multiport Switch2/2
  Constant16/1 -> Multiport Switch2/3
  Constant17/1 -> Multiport Switch2/4
  Constant18/1 -> Multiport Switch2/5
  Constant27/1 -> Multiport Switch2/6
  Constant28/1 -> Multiport Switch2/7
  Divide/1 -> Output/1
  Multiport Switch2/1 -> HwModeRegister/1
  Product_out_dtc/1 -> Divide/1
  PipelineRegister/1 -> Product_out_dtc/1
  Product/1 -> PipelineRegister/1
  HwModeRegister/1 -> Product/1
  HwModeRegister1/1 -> Product/2

== system gm_UZ_EnDat/UZ_ENDAT/DIFFBUILDER ==
  DATAT0 : Inport  OutDataTypeStr=uint32  PortDimensions=1
  DATAT1 : Inport  Port=2  OutDataTypeStr=uint32  PortDimensions=1
  DATAT2 : Inport  Port=3  OutDataTypeStr=uint32  PortDimensions=1
  Trigger : TriggerPort  VariantControl=(inherit)  OutputDataType=int8  InitialTriggerSignalState=positive  PortDimensions=1  OutDataTypeStr=boolean
  Subtract : Sum  Inputs=+-  OutDataTypeStr=int32  AccumDataTypeStr=fixdt(1, 33, 0)  RndMeth=Simplest  SaturateOnIntegerOverflow=on
  Subtract1 : Sum  Inputs=+-  OutDataTypeStr=int32  AccumDataTypeStr=fixdt(1, 33, 0)  RndMeth=Simplest  SaturateOnIntegerOverflow=on
  DIFT1T0 : Outport  InitialOutput=0
  DIFT2T0 : Outport  Port=2  InitialOutput=0
  wires:
  DATAT0/1 -> Subtract1/1, Subtract/1
  DATAT1/1 -> Subtract/2
  DATAT2/1 -> Subtract1/2
  Subtract/1 -> DIFT1T0/1
  Subtract1/1 -> DIFT2T0/1

== system gm_UZ_EnDat/UZ_ENDAT/Detect Change ==
  note: U(k)
  note: Edge
  U : Inport  OutDataTypeStr=fixdt(0, 4, 0)  SampleTime=1e-08
  Delay Input1 : Delay  DelayLength=double(1)  InitialCondition=0  SampleTime=1e-08
  FixPt Relational Operator : RelationalOperator  Operator=~=  OutDataTypeStr=boolean  SampleTime=1e-08  InputSameDT=off
  Y : Outport  SampleTime=1e-08
  wires:
  U/1 -> FixPt Relational Operator/1, Delay Input1/1
  Delay Input1/1 -> FixPt Relational Operator/2
  FixPt Relational Operator/1 -> Y/1

== system gm_UZ_EnDat/UZ_ENDAT/INITIALOFF ==
  CLKAUX : Inport  OutDataTypeStr=boolean  PortDimensions=1  SampleTime=1e-08
  CLK : Inport  Port=2  OutDataTypeStr=boolean  PortDimensions=1  SampleTime=1e-08
  DATAWR : Inport  Port=3  OutDataTypeStr=boolean  PortDimensions=1  SampleTime=1e-08
  DATA : Inport  Port=4  OutDataTypeStr=boolean  PortDimensions=1  SampleTime=1e-08
  CLKWR : Inport  Port=5  OutDataTypeStr=boolean  PortDimensions=1  SampleTime=1e-08
  FACTOR : Inport  Port=6  OutDataTypeStr=uint16  PortDimensions=1  SampleTime=1e-08
  CLKCNTER_FAST : Subsystem
  Constant : Constant  Value=0  OutDataTypeStr=boolean  SampleTime=1e-08
  Multiport Switch{,1..3} (4 alike) : MultiPortSwitch  DataPortOrder=Zero-based contiguous  Inputs=2  DiagnosticForDefault=None  zeroidx=on  SampleTime=1e-08  SaturateOnIntegerOverflow=off  InputSameDT=off
  Relational Operator : RelationalOperator  Operator=<  OutDataTypeStr=boolean  SampleTime=1e-08  InputSameDT=off
  Subsystem6 : Subsystem
  rd_0 : Delay  DelayLength=double(3)  InitialCondition=0  SampleTime=1e-08
  rd_1 : Delay  DelayLength=double(1)  InitialCondition=0  SampleTime=1e-08
  rd_2 : Delay  DelayLength=double(1)  InitialCondition=0  SampleTime=1e-08
  CLK_OUT : Outport  SampleTime=1e-08
  DATAWR_OUT : Outport  Port=2  SampleTime=1e-08
  DATA_OUT : Outport  Port=3  SampleTime=1e-08
  CLKWR_OUT : Outport  Port=4  SampleTime=1e-08
  wires:
  CLKAUX/1 -> CLKCNTER_FAST/1(CLK)
  CLK/1 -> Multiport Switch/2
  DATAWR/1 -> Multiport Switch1/2
  DATA/1 -> rd_2/1
  CLKWR/1 -> Multiport Switch3/2
  FACTOR/1 -> Subsystem6/1(FACTOR)
  Constant/1 -> Multiport Switch3/3, Multiport Switch2/3, Multiport Switch1/3, Multiport Switch/3
  Multiport Switch/1 -> CLK_OUT/1
  Multiport Switch1/1 -> DATAWR_OUT/1
  Multiport Switch2/1 -> DATA_OUT/1
  Multiport Switch3/1 -> CLKWR_OUT/1
  Relational Operator/1 -> rd_1/1, Multiport Switch3/1, Multiport Switch1/1, Multiport Switch/1
  Subsystem6/1(out) -> Relational Operator/2
  CLKCNTER_FAST/1(CNT) -> rd_0/1
  rd_0/1 -> Relational Operator/1
  rd_2/1 -> Multiport Switch2/2
  rd_1/1 -> Multiport Switch2/1

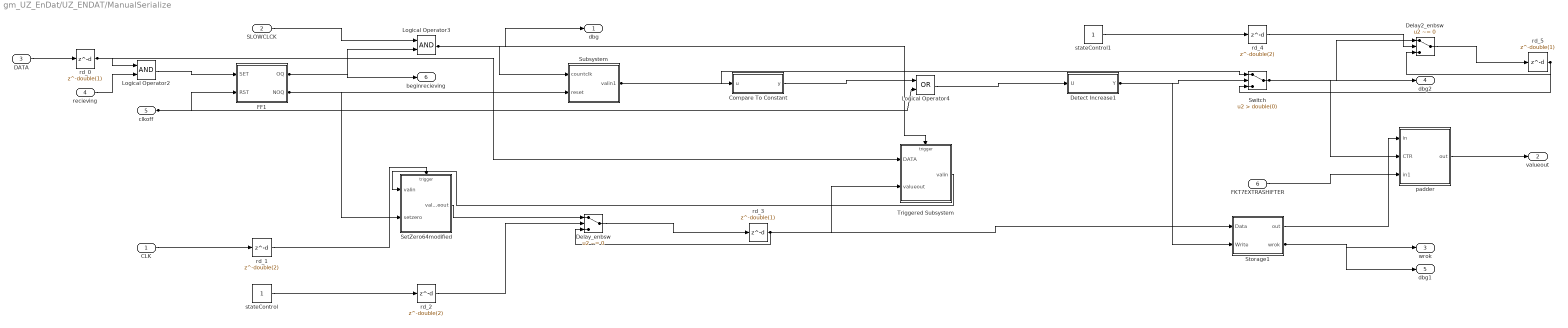
== system gm_UZ_EnDat/UZ_ENDAT/ManualSerialize ==
  CLK : Inport  OutDataTypeStr=boolean  PortDimensions=1  SampleTime=1e-08
  SLOWCLCK : Inport  Port=2  OutDataTypeStr=boolean  PortDimensions=1  SampleTime=1e-08
  DATA : Inport  Port=3  OutDataTypeStr=boolean  PortDimensions=1  SampleTime=1e-08
  recieving : Inport  Port=4  OutMin=0  OutMax=1  OutDataTypeStr=boolean  PortDimensions=1  SampleTime=1e-08
  clkoff : Inport  Port=5  OutMin=0  OutMax=1  OutDataTypeStr=boolean  PortDimensions=1  SampleTime=1e-08
  FKT7EXTRASHIFTER : Inport  Port=6  OutDataTypeStr=int8  PortDimensions=1  SampleTime=1e-08
  Compare To Constant : Subsystem  mask(Compare To Constant){relop===, const=double(48), OutDataTypeStr=boolean, ZeroCross=on}
      mask prompts: relop "Simulink:masks:Operator_MP"; const "Simulink:masks:ConstantValue_MP"; OutDataTypeStr "Simulink:masks:OutputDataType_MP"; ZeroCross "Simulink:masks:EnableZerocrossingDetection_MP"
      mask help: Simulink:masks:CompareToConstant_MD
      mask init:
      | OutDataTypeStr = 'boolean';
      | ZeroCross = 'on';
      | blkName = 'UZ_EnDat/UZ_ENDAT/ManualSerialize/Compare\nTo Constant';
      | const = double(48);
      | const_str = '48';
      | const_val = double(48);
      | relop = '==';
      | setValue = 'boolean';
      | str = '== 48';
      mask TypeOptions relop: == | ~= | < | <= | >= | >
      mask TypeOptions OutDataTypeStr: Simulink:masks:uint8 | Simulink:masks:boolean
      mask Callback ZeroCross: sl('zeroCrossEnable', gcbh);
      mask Display: disp(str)
  Delay2_enbsw : Switch  Criteria=u2 ~= 0  Threshold=double(0)  OutDataTypeStr=uint8  SampleTime=1e-08  SaturateOnIntegerOverflow=off  InputSameDT=off
  Delay_enbsw : Switch  Criteria=u2 ~= 0  Threshold=double(0)  OutDataTypeStr=fixdt(0, 64, 0)  SampleTime=1e-08  SaturateOnIntegerOverflow=off  InputSameDT=off
  Detect Increase1 : Subsystem  mask(Detect Increase){vinit=double(0), InputProcessing=Elements as channels (sample based), OutDataTypeStr=boolean}
      mask prompts: vinit "Simulink:masks:InitialCondition_MP"; InputProcessing "Simulink:masks:InputProcessing_MP"; OutDataTypeStr "Simulink:masks:OutputDataType_MP"
      mask help: Simulink:masks:DetectIncrease_MD
      mask TypeOptions InputProcessing: Simulink:masks:ColumnsAsChannelsFrameBased | Simulink:masks:ElementsAsChannelsSampleBased
      mask TypeOptions OutDataTypeStr: Simulink:masks:uint8 | Simulink:masks:boolean
      mask Display: fprintf('U > U/z')
  FF1 : Subsystem
  Logical Operator2 : Logic  AllPortsSameDT=off  OutDataTypeStr=boolean  SampleTime=1e-08
  Logical Operator3 : Logic  AllPortsSameDT=off  OutDataTypeStr=boolean  SampleTime=1e-08
  Logical Operator4 : Logic  Operator=OR  AllPortsSameDT=off  OutDataTypeStr=boolean  SampleTime=1e-08
  SetZero64modified : Subsystem
  Storage1 : Subsystem
  Subsystem : Subsystem
  Switch : Switch  Criteria=u2 > Threshold  Threshold=double(0)  OutDataTypeStr=uint8  SampleTime=1e-08  SaturateOnIntegerOverflow=off  InputSameDT=off
  Triggered Subsystem : Subsystem
  padder : Subsystem
  rd_0 : Delay  DelayLength=double(1)  InitialCondition=0  SampleTime=1e-08
  rd_1 : Delay  DelayLength=double(2)  InitialCondition=0  SampleTime=1e-08
  rd_2 : Delay  DelayLength=double(2)  InitialCondition=0  SampleTime=1e-08
  rd_3 : Delay  DelayLength=double(1)  InitialCondition=0  SampleTime=1e-08
  rd_4 : Delay  DelayLength=double(2)  InitialCondition=0  SampleTime=1e-08
  rd_5 : Delay  DelayLength=double(1)  InitialCondition=0  SampleTime=1e-08
  stateControl : Constant  OutDataTypeStr=boolean  SampleTime=1e-08
  stateControl1 : Constant  OutDataTypeStr=boolean  SampleTime=1e-08
  dbg : Outport  OutDataTypeStr=boolean  SampleTime=1e-08  VectorParamsAs1DForOutWhenUnconnected=off
  valueout : Outport  Port=2  OutDataTypeStr=uint64  SampleTime=1e-08
  wrok : Outport  Port=3  OutDataTypeStr=boolean  SampleTime=1e-08
  dbg2 : Outport  Port=4  OutDataTypeStr=uint8  SampleTime=1e-08  VectorParamsAs1DForOutWhenUnconnected=off
  dbg1 : Outport  Port=5  OutDataTypeStr=boolean  SampleTime=1e-08  VectorParamsAs1DForOutWhenUnconnected=off
  beginrecieving : Outport  Port=6  OutDataTypeStr=boolean  SampleTime=1e-08  VectorParamsAs1DForOutWhenUnconnected=off
  wires:
  SLOWCLCK/1 -> Logical Operator3/1
  recieving/1 -> Logical Operator2/2
  clkoff/1 -> Logical Operator4/2, FF1/2(RST)
  FKT7EXTRASHIFTER/1 -> padder/3(in1)
  Compare To Constant/1(y) -> Logical Operator4/1
  Detect Increase1/1(Y) -> Storage1/2(Write), Switch/2
  FF1/1(OQ) -> Logical Operator3/2, beginrecieving/1
  FF1/2(NOQ) -> Subsystem/2(reset), SetZero64modified/2(setzero)
  Logical Operator2/1 -> FF1/1(SET)
  Logical Operator3/1 -> dbg/1, Subsystem/1(countclk), Triggered Subsystem/Trigger
  Logical Operator4/1 -> Detect Increase1/1(U)
  Storage1/1(out) -> padder/1(in)
  Storage1/2(wrok) -> dbg1/1, wrok/1
  Subsystem/1(valin1) -> Compare To Constant/1(u), Switch/1
  padder/1(out) -> valueout/1
  CLK/1 -> rd_1/1
  stateControl/1 -> rd_2/1
  stateControl1/1 -> rd_4/1
  Switch/1 -> Delay2_enbsw/1, dbg2/1, padder/2(CTR)
  Triggered Subsystem/1(valin) -> SetZero64modified/1(valin)
  SetZero64modified/1(valueout) -> Delay_enbsw/1
  rd_2/1 -> Delay_enbsw/2
  rd_4/1 -> Delay2_enbsw/2
  rd_1/1 -> SetZero64modified/Trigger
  DATA/1 -> rd_0/1
  rd_0/1 -> Logical Operator2/1, Triggered Subsystem/1(DATA)
  Delay_enbsw/1 -> rd_3/1
  rd_3/1 -> Delay_enbsw/3, Triggered Subsystem/2(valueout), Storage1/1(Data)
  Delay2_enbsw/1 -> rd_5/1
  rd_5/1 -> Delay2_enbsw/3, Switch/3

== system gm_UZ_EnDat/UZ_ENDAT/OUTPUTCONTROLCONTINIOUS ==
  CLKCNT : Inport  OutDataTypeStr=uint32  PortDimensions=1  SampleTime=1e-08
  CLKS2DATAFLOWCHG : Inport  Port=2  OutDataTypeStr=uint16  PortDimensions=1  SampleTime=1e-08
  CLK2ENDOFTRANSMISSION : Inport  Port=3  OutDataTypeStr=uint16  PortDimensions=1  SampleTime=1e-08
  OPENCOM : Inport  Port=4  OutDataTypeStr=boolean  PortDimensions=1  SampleTime=1e-08
  CLKCNTNOSTOP : Inport  Port=5  OutDataTypeStr=uint32  PortDimensions=1  SampleTime=1e-08
  RECOVERYTIME : Inport  Port=6  OutDataTypeStr=uint16  PortDimensions=1  SampleTime=1e-08
  Add : Sum  OutDataTypeStr=uint16  AccumDataTypeStr=uint16  SampleTime=1e-08
  Constant : Constant  Value=0  OutDataTypeStr=uint8  SampleTime=1e-08
  Logical Operator : Logic  Operator=OR  AllPortsSameDT=off  OutDataTypeStr=boolean  SampleTime=1e-08
  Logical Operator1 : Logic  AllPortsSameDT=off  OutDataTypeStr=boolean  SampleTime=1e-08
  Logical Operator6 : Logic  Operator=NOT  Inputs=1  AllPortsSameDT=off  OutDataTypeStr=boolean  SampleTime=1e-08
  Relational Operator : RelationalOperator  Operator=<=  OutDataTypeStr=boolean  SampleTime=1e-08  InputSameDT=off
  Relational Operator1 : RelationalOperator  OutDataTypeStr=boolean  SampleTime=1e-08  InputSameDT=off
  Relational Operator2 : RelationalOperator  OutDataTypeStr=boolean  SampleTime=1e-08  InputSameDT=off
  Relational Operator3 : RelationalOperator  OutDataTypeStr=boolean  SampleTime=1e-08  InputSameDT=off
  CLKOFF : Outport  OutDataTypeStr=boolean  SampleTime=1e-08
  DATAINV : Outport  Port=2  OutDataTypeStr=boolean  SampleTime=1e-08
  RESETCNT : Outport  Port=3  OutDataTypeStr=boolean  SampleTime=1e-08
  wires:
  CLKCNT/1 -> Relational Operator2/1, Relational Operator1/1, Relational Operator/1
  CLKS2DATAFLOWCHG/1 -> Relational Operator/2
  CLK2ENDOFTRANSMISSION/1 -> Relational Operator1/2, Add/1
  OPENCOM/1 -> Logical Operator6/1
  CLKCNTNOSTOP/1 -> Relational Operator3/1
  RECOVERYTIME/1 -> Add/2
  Add/1 -> Relational Operator3/2
  Logical Operator/1 -> CLKOFF/1
  Logical Operator1/1 -> DATAINV/1
  Logical Operator6/1 -> Logical Operator/1
  Relational Operator/1 -> Logical Operator1/1
  Relational Operator1/1 -> Logical Operator/2
  Relational Operator2/1 -> Logical Operator1/2
  Relational Operator3/1 -> RESETCNT/1
  Constant/1 -> Relational Operator2/2

== system gm_UZ_EnDat/UZ_ENDAT/RECOVERYTIMESELECTOR ==
  In1 : Inport  OutDataTypeStr=fixdt(0, 4, 0)  PortDimensions=1  SampleTime=1e-08
  FAKTOR : Inport  Port=2  OutDataTypeStr=uint16  PortDimensions=1  SampleTime=1e-08
  Constant : Constant  Value=100  OutDataTypeStr=uint16  SampleTime=1e-08
  Constant19 : Constant  Value=96  OutDataTypeStr=uint16  SampleTime=1e-08
  Constant20 : Constant  Value=48  OutDataTypeStr=uint16  SampleTime=1e-08
  Constant21 : Constant  Value=192  OutDataTypeStr=uint16  SampleTime=1e-08
  Constant22 : Constant  Value=255  OutDataTypeStr=uint16  SampleTime=1e-08
  Constant25 : Constant  Value=24  OutDataTypeStr=uint16  SampleTime=1e-08
  Constant26 : Constant  Value=12  OutDataTypeStr=uint16  SampleTime=1e-08
  Constant5 : Constant  Value=6  OutDataTypeStr=uint16  SampleTime=1e-08
  Divide : Product  Inputs=*/  OutDataTypeStr=uint16  RndMeth=Simplest  SaturateOnIntegerOverflow=on  SampleTime=1e-08
  HwModeRegister : Delay  DelayLength=double(1)  InitialCondition=0  SampleTime=1e-08
  HwModeRegister1 : Delay  DelayLength=double(1)  InitialCondition=0  SampleTime=1e-08
  Multiport Switch3 : MultiPortSwitch  DataPortOrder=Zero-based contiguous  Inputs=7  DiagnosticForDefault=None  zeroidx=on  OutDataTypeStr=uint16  SampleTime=1e-08  SaturateOnIntegerOverflow=off  InputSameDT=off
  PipelineRegister : Delay  DelayLength=double(1)  InitialCondition=0  SampleTime=1e-08
  Product : Product  Inputs=**  OutDataTypeStr=uint32  SampleTime=1e-08
  Product_out_dtc : DataTypeConversion  OutDataTypeStr=uint16  RndMeth=Simplest  SampleTime=1e-08
  Out1 : Outport  SampleTime=1e-08
  wires:
  In1/1 -> Multiport Switch3/1
  FAKTOR/1 -> HwModeRegister1/1
  Constant/1 -> Divide/2
  Constant19/1 -> Multiport Switch3/4
  Constant20/1 -> Multiport Switch3/5
  Constant21/1 -> Multiport Switch3/3
  Constant22/1 -> Multiport Switch3/2
  Constant25/1 -> Multiport Switch3/6
  Constant26/1 -> Multiport Switch3/7
  Constant5/1 -> Multiport Switch3/8
  Divide/1 -> Out1/1
  Multiport Switch3/1 -> HwModeRegister/1
  Product_out_dtc/1 -> Divide/1
  PipelineRegister/1 -> Product_out_dtc/1
  Product/1 -> PipelineRegister/1
  HwModeRegister/1 -> Product/1
  HwModeRegister1/1 -> Product/2
